simulink model "sldemo_clutch"  (R2020b)
settings: Solver=VariableStepAuto  StartTime=0.0  StopTime=10.0  RelTol=1e-3
PostLoadFcn:
  | sldemo_clutchplot
StartFcn:
  | sldemo_clutchplot Start
StopFcn:
  | if exist ('sldemo_clutch_output')
  |    sldemo_clutchplot Stop
  | end
values from neighbouring files (symbols this model uses):
  be = 2.0    [Clutch_Data_Dict.sldd]
  bv = 1.0    [Clutch_Data_Dict.sldd]
  Ie = 1.0    [Clutch_Data_Dict.sldd]
  Iv = 5.0    [Clutch_Data_Dict.sldd]
  muk = 1.0    [Clutch_Data_Dict.sldd]
  mus = 1.5    [Clutch_Data_Dict.sldd]
  R = 1.0    [Clutch_Data_Dict.sldd]
CloseFcn:
  | sldemo_clutchplot Close
settings Model: DataDictionary=Clutch_Data_Dict.sldd  Creator=vijay jagtap  LastModifiedBy=vijay jagtap
settings SolverCC: ZeroCrossAlgorithm=Adaptive
settings DebuggingCC: IgnoredZcDiagnostic=none

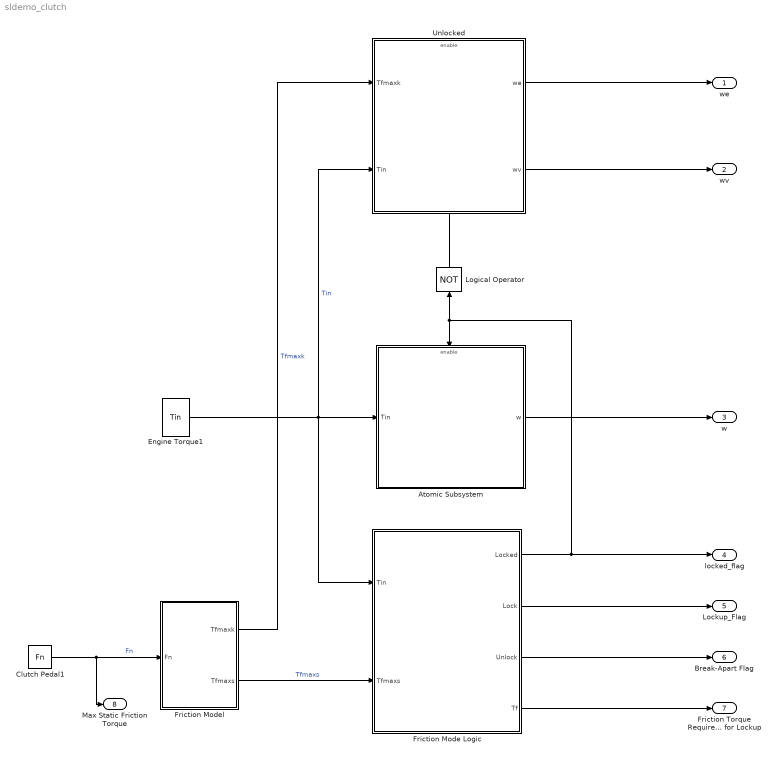
== system sldemo_clutch ==
  Atomic Subsystem : Subsystem  TreatAsAtomicUnit=on
  Clutch Pedal1 : FromWorkspace  VariableName=Fn  ZeroCross=off
  Engine Torque1 : FromWorkspace  VariableName=Tin  ZeroCross=off
  Friction Model : Subsystem
  Friction Mode Logic : Subsystem
  Logical Operator : Logic  Operator=NOT  AllPortsSameDT=off  OutDataTypeStr=boolean
  Unlocked : Subsystem  TreatAsAtomicUnit=on
  we : Outport
  wv : Outport  Port=2
  w : Outport  Port=3
  locked_flag : Outport  Port=4
  Lockup_Flag : Outport  Port=5
  Break-Apart Flag : Outport  Port=6
  Friction Torque Required for Lockup : Outport  Port=7
  Max Static Friction Torque : Outport  Port=8
  wires:
  Clutch Pedal1/1 -> Max Static Friction Torque/1, Friction Model/1(Fn)  "Fn"
  Friction Model/2(Tfmaxs) -> Friction Mode Logic/2(Tfmaxs)  "Tfmaxs"
  Engine Torque1/1 -> Unlocked/2(Tin), Friction Mode Logic/1(Tin), Atomic Subsystem/1(Tin)  "Tin"
  Friction Model/1(Tfmaxk) -> Unlocked/1(Tfmaxk)  "Tfmaxk"
  Friction Mode Logic/1(Locked) -> Logical Operator/1, Atomic Subsystem/Enable, locked_flag/1
  Friction Mode Logic/2(Lock) -> Lockup_Flag/1
  Friction Mode Logic/3(Unlock) -> Break-Apart Flag/1
  Friction Mode Logic/4(Tf) -> Friction Torque Required for Lockup/1
  Atomic Subsystem/1(w) -> w/1
  Unlocked/2(wv) -> wv/1
  Unlocked/1(we) -> we/1
  Logical Operator/1 -> Unlocked/Enable

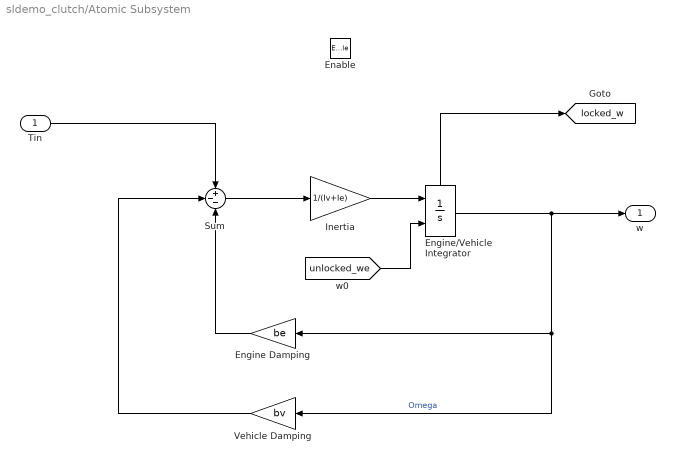
== system sldemo_clutch/Atomic Subsystem ==
  Tin : Inport
  Enable : EnablePort  StatesWhenEnabling=reset
  Engine Damping : Gain  Gain=be  SaturateOnIntegerOverflow=on  OutDataTypeStr=Inherit: Same as input  ParamDataTypeStr=Inherit: Same as input
  Engine/Vehicle Integrator : Integrator  InitialConditionSource=external  ShowStatePort=on
  Inertia : Gain  Gain=1/(Iv+Ie)  SaturateOnIntegerOverflow=on  OutDataTypeStr=Inherit: Same as input  ParamDataTypeStr=Inherit: Same as input
  Sum : Sum  Inputs=+--  InputSameDT=on  SaturateOnIntegerOverflow=on  OutDataTypeStr=Inherit: Same as first input
  Vehicle Damping : Gain  Gain=bv  SaturateOnIntegerOverflow=on  OutDataTypeStr=Inherit: Same as input  ParamDataTypeStr=Inherit: Same as input
  w : Outport  InitialOutput=0  VectorParamsAs1DForOutWhenUnconnected=off
  tag scope: locked_w=global
  wires:
  Inertia/1 -> Engine/Vehicle Integrator/1
  Engine Damping/1 -> Sum/3
  Vehicle Damping/1 -> Sum/2
  Tin/1 -> Sum/1
  Engine/Vehicle Integrator/1 -> Engine Damping/1, Vehicle Damping/1, w/1  "Omega"
  Engine/Vehicle Integrator/State -> [locked_w]
  [unlocked_we] -> Engine/Vehicle Integrator/2
  Sum/1 -> Inertia/1

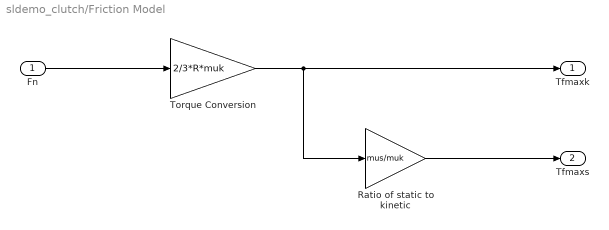
== system sldemo_clutch/Friction Model ==
  Fn : Inport
  Ratio of static to kinetic : Gain  Gain=mus/muk  SaturateOnIntegerOverflow=on  OutDataTypeStr=Inherit: Same as input  ParamDataTypeStr=Inherit: Same as input
  Torque Conversion : Gain  Gain=2/3*R*muk  SaturateOnIntegerOverflow=on  OutDataTypeStr=Inherit: Same as input  ParamDataTypeStr=Inherit: Same as input
  Tfmaxk : Outport  InitialOutput=0  VectorParamsAs1DForOutWhenUnconnected=off
  Tfmaxs : Outport  Port=2  InitialOutput=0  VectorParamsAs1DForOutWhenUnconnected=off
  wires:
  Torque Conversion/1 -> Tfmaxk/1, Ratio of static to kinetic/1
  Fn/1 -> Torque Conversion/1
  Ratio of static to kinetic/1 -> Tfmaxs/1

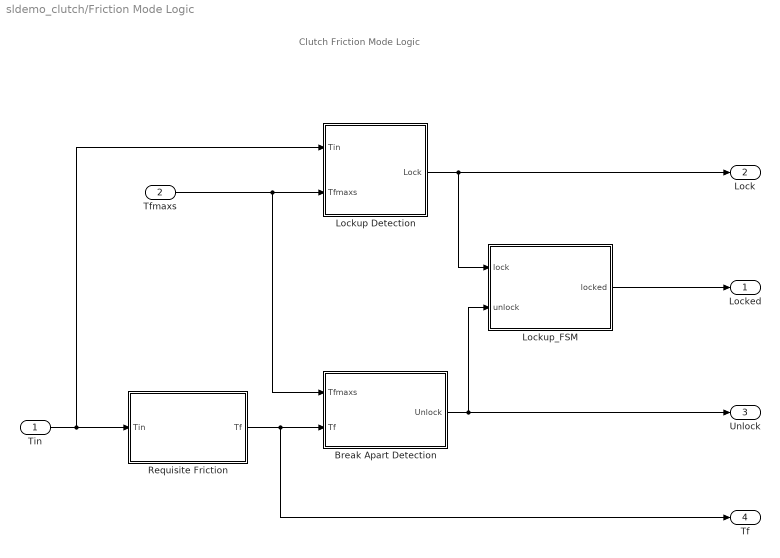
== system sldemo_clutch/Friction Mode Logic ==
  note: Clutch Friction Mode Logic
  Tin : Inport
  Tfmaxs : Inport  Port=2
  Break Apart Detection : Subsystem
  Lockup Detection : Subsystem
  Lockup_FSM : Subsystem
  Requisite Friction : Subsystem
  Locked : Outport
  Lock : Outport  Port=2
  Unlock : Outport  Port=3
  Tf : Outport  Port=4
  wires:
  Requisite Friction/1(Tf) -> Tf/1, Break Apart Detection/2(Tf)
  Break Apart Detection/1(Unlock) -> Lockup_FSM/2(unlock), Unlock/1
  Lockup Detection/1(Lock) -> Lockup_FSM/1(lock), Lock/1
  Tin/1 -> Lockup Detection/1(Tin), Requisite Friction/1(Tin)
  Tfmaxs/1 -> Break Apart Detection/1(Tfmaxs), Lockup Detection/2(Tfmaxs)
  Lockup_FSM/1(locked) -> Locked/1

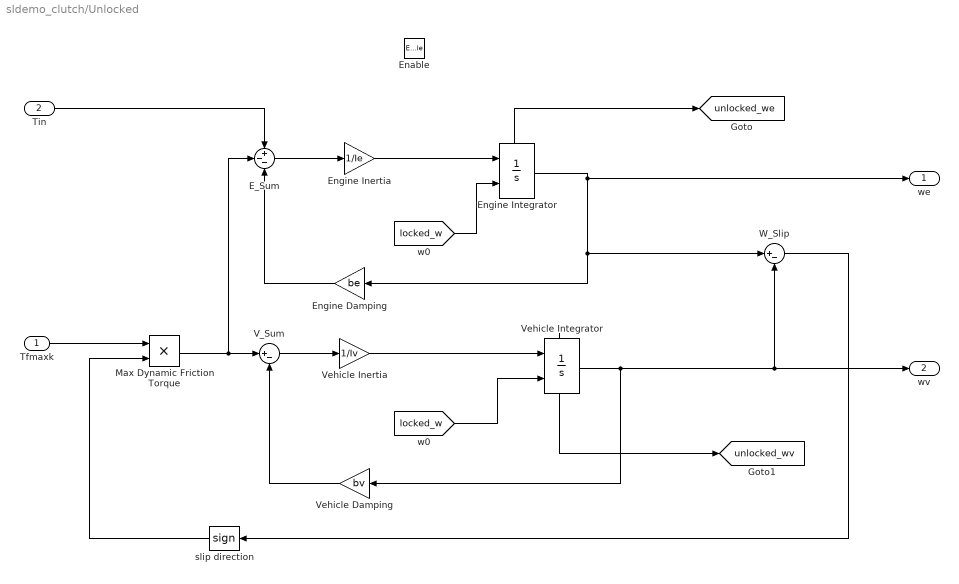
== system sldemo_clutch/Unlocked ==
  Tfmaxk : Inport
  Tin : Inport  Port=2
  Enable : EnablePort  StatesWhenEnabling=reset
  E_Sum : Sum  Inputs=+--  InputSameDT=on  SaturateOnIntegerOverflow=on  OutDataTypeStr=Inherit: Same as first input
  Engine Damping : Gain  Gain=be  SaturateOnIntegerOverflow=on  OutDataTypeStr=Inherit: Same as input  ParamDataTypeStr=Inherit: Same as input
  Engine Inertia : Gain  Gain=1/Ie  SaturateOnIntegerOverflow=on  OutDataTypeStr=Inherit: Same as input  ParamDataTypeStr=Inherit: Same as input
  Engine Integrator : Integrator  InitialConditionSource=external  ShowStatePort=on
  Max Dynamic Friction Torque : Product  InputSameDT=on  RndMeth=Zero  SaturateOnIntegerOverflow=on  OutDataTypeStr=Inherit: Same as first input
  V_Sum : Sum  Inputs=|+-  InputSameDT=on  SaturateOnIntegerOverflow=on  OutDataTypeStr=Inherit: Same as first input
  Vehicle Damping : Gain  Gain=bv  SaturateOnIntegerOverflow=on  OutDataTypeStr=Inherit: Same as input  ParamDataTypeStr=Inherit: Same as input
  Vehicle Inertia : Gain  Gain=1/Iv  SaturateOnIntegerOverflow=on  OutDataTypeStr=Inherit: Same as input  ParamDataTypeStr=Inherit: Same as input
  Vehicle Integrator : Integrator  InitialConditionSource=external  ShowStatePort=on
  W_Slip : Sum  Inputs=|+-  InputSameDT=on  SaturateOnIntegerOverflow=on  OutDataTypeStr=Inherit: Same as first input
  slip direction : Signum
  we : Outport  InitialOutput=0  VectorParamsAs1DForOutWhenUnconnected=off
  wv : Outport  Port=2  InitialOutput=0  VectorParamsAs1DForOutWhenUnconnected=off
  tag scope: unlocked_we=global, unlocked_wv=global
  wires:
  W_Slip/1 -> slip direction/1
  Engine Inertia/1 -> Engine Integrator/1
  Engine Integrator/1 -> we/1, Engine Damping/1, W_Slip/1
  Tfmaxk/1 -> Max Dynamic Friction Torque/1
  Vehicle Integrator/1 -> wv/1, W_Slip/2, Vehicle Damping/1
  Vehicle Inertia/1 -> Vehicle Integrator/1
  slip direction/1 -> Max Dynamic Friction Torque/2
  Vehicle Integrator/State -> [unlocked_wv]
  [locked_w] -> Vehicle Integrator/2
  Engine Integrator/State -> [unlocked_we]
  V_Sum/1 -> Vehicle Inertia/1
  [locked_w] -> Engine Integrator/2
  E_Sum/1 -> Engine Inertia/1
  Vehicle Damping/1 -> V_Sum/2
  Tin/1 -> E_Sum/1
  Max Dynamic Friction Torque/1 -> V_Sum/1, E_Sum/2
  Engine Damping/1 -> E_Sum/3

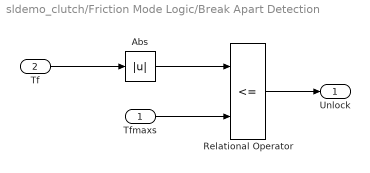
== system sldemo_clutch/Friction Mode Logic/Break Apart Detection ==
  Tfmaxs : Inport
  Tf : Inport  Port=2
  Abs : Abs
  Relational Operator : RelationalOperator  Operator=<=  OutDataTypeStr=boolean  RndMeth=Simplest
  Unlock : Outport
  wires:
  Abs/1 -> Relational Operator/1
  Tfmaxs/1 -> Relational Operator/2
  Tf/1 -> Abs/1
  Relational Operator/1 -> Unlock/1

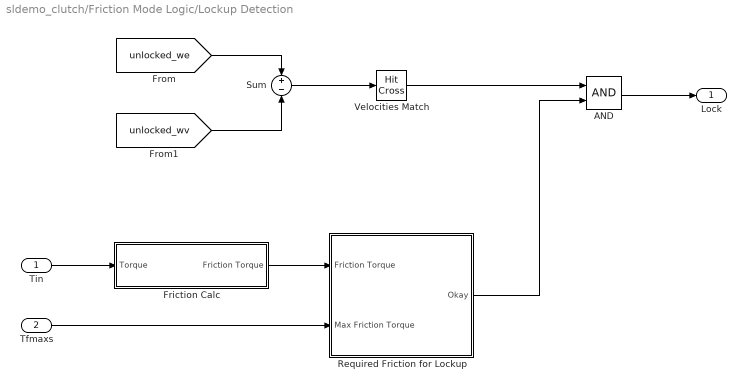
== system sldemo_clutch/Friction Mode Logic/Lockup Detection ==
  Tin : Inport
  Tfmaxs : Inport  Port=2
  AND : Logic  AllPortsSameDT=off  OutDataTypeStr=boolean
  Friction Calc : Subsystem
  Required Friction for Lockup : Subsystem
  Sum : Sum  Inputs=+-
  Velocities Match : HitCross
  Lock : Outport
  wires:
  Friction Calc/1(Friction Torque) -> Required Friction for Lockup/1(Friction Torque)
  [unlocked_we] -> Sum/1
  [unlocked_wv] -> Sum/2
  Tin/1 -> Friction Calc/1(Torque)
  Tfmaxs/1 -> Required Friction for Lockup/2(Max Friction Torque)
  Sum/1 -> Velocities Match/1
  Velocities Match/1 -> AND/1
  Required Friction for Lockup/1(Okay) -> AND/2
  AND/1 -> Lock/1

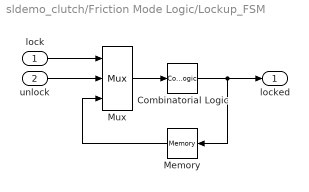
== system sldemo_clutch/Friction Mode Logic/Lockup_FSM ==
  lock : Inport
  unlock : Inport  Port=2
  Combinatorial Logic : CombinatorialLogic  TruthTable=[0;1;0;0;1;1;1;0]
  Memory : Memory
  Mux : Mux  Inputs=3
  locked : Outport  InitialOutput=0  VectorParamsAs1DForOutWhenUnconnected=off
  wires:
  lock/1 -> Mux/1
  Mux/1 -> Combinatorial Logic/1
  Combinatorial Logic/1 -> locked/1, Memory/1
  Memory/1 -> Mux/3
  unlock/1 -> Mux/2

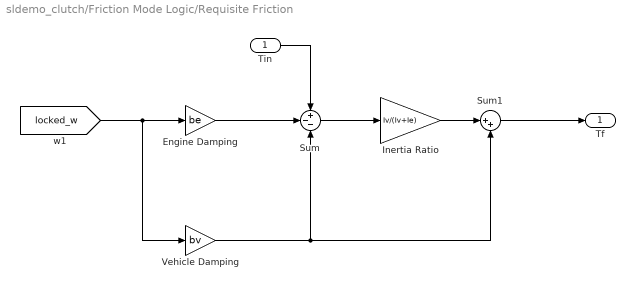
== system sldemo_clutch/Friction Mode Logic/Requisite Friction ==
  Tin : Inport
  Engine Damping : Gain  Gain=be
  Inertia Ratio : Gain  Gain=Iv/(Iv+Ie)
  Sum : Sum  Inputs=+--
  Sum1 : Sum  Inputs=|++
  Vehicle Damping : Gain  Gain=bv
  Tf : Outport
  wires:
  Vehicle Damping/1 -> Sum1/2, Sum/3
  Engine Damping/1 -> Sum/2
  Tin/1 -> Sum/1
  [locked_w] -> Vehicle Damping/1, Engine Damping/1
  Sum1/1 -> Tf/1
  Inertia Ratio/1 -> Sum1/1
  Sum/1 -> Inertia Ratio/1

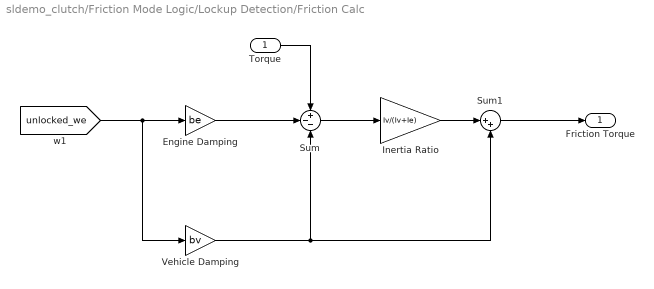
== system sldemo_clutch/Friction Mode Logic/Lockup Detection/Friction Calc ==
  Torque : Inport
  Engine Damping : Gain  Gain=be
  Inertia Ratio : Gain  Gain=Iv/(Iv+Ie)
  Sum : Sum  Inputs=+--
  Sum1 : Sum  Inputs=|++
  Vehicle Damping : Gain  Gain=bv
  Friction Torque : Outport
  wires:
  Engine Damping/1 -> Sum/2
  Sum/1 -> Inertia Ratio/1
  [unlocked_we] -> Vehicle Damping/1, Engine Damping/1
  Vehicle Damping/1 -> Sum1/2, Sum/3
  Torque/1 -> Sum/1
  Inertia Ratio/1 -> Sum1/1
  Sum1/1 -> Friction Torque/1

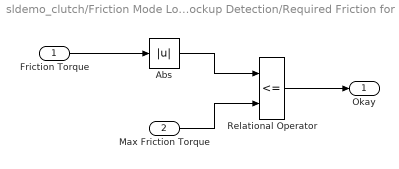
== system sldemo_clutch/Friction Mode Logic/Lockup Detection/Required Friction for Lockup ==
  Friction Torque : Inport
  Max Friction Torque : Inport  Port=2
  Abs : Abs  SaturateOnIntegerOverflow=on
  Relational Operator : RelationalOperator  Operator=<=  OutDataTypeStr=boolean  RndMeth=Nearest
  Okay : Outport
  wires:
  Abs/1 -> Relational Operator/1
  Friction Torque/1 -> Abs/1
  Max Friction Torque/1 -> Relational Operator/2
  Relational Operator/1 -> Okay/1
